simulink model "adcs_v15_integral_Power_dist"  (Simulink 7.4)
settings: Solver=ode4  StartTime=0.0  StopTime=120000  FixedStep=s_SIM_STEP_SIZE  RelTol=1e-3
values from neighbouring files (symbols this model uses):
  A = ((T_SIDE + .29)*1e-3)^2    [constants_v13.m]    (also in constants_v15.m; constants_v15_Pow.m; constants_v15_Pow_ss_error.m; constants_v16_integral_kartavya.m)
  AMP = 4e-8    (= 4e-08)    [constants_v15_Pow.m]
  Area_SP_S1 = 4*11*0.02025*0.04025    (= 0.03586275)    [constants_v15_Pow.m]    (also in constants_v15_Pow_ss_error.m; constants_v16_integral_light_sun_sgp_igrf_power_13Dec2011.m)
  Area_SP_S2 = 4*11*0.02025*0.04025    (= 0.03586275)    [constants_v15_Pow.m]    (also in constants_v15_Pow_ss_error.m; constants_v16_integral_light_sun_sgp_igrf_power_13Dec2011.m)
  Area_SP_S3 = 0.0    (= 0)    [constants_v15_Pow.m]    (also in constants_v15_Pow_ss_error.m; constants_v16_integral_light_sun_sgp_igrf_power_13Dec2011.m)
  Area_SP_S4 = 4*11*0.02025*0.04025    (= 0.03586275)    [constants_v15_Pow.m]    (also in constants_v15_Pow_ss_error.m; constants_v16_integral_light_sun_sgp_igrf_power_13Dec2011.m)
  Area_SP_S5 = 0.0    (= 0)    [constants_v15_Pow.m]    (also in constants_v15_Pow_ss_error.m; constants_v16_integral_light_sun_sgp_igrf_power_13Dec2011.m)
  Area_SP_S6 = 3*11*0.02025*0.04025    (= 0.0268970625)    [constants_v15_Pow.m]    (also in constants_v15_Pow_ss_error.m; constants_v16_integral_light_sun_sgp_igrf_power_13Dec2011.m)
  Ca_Solar_Drag = 1.4    [constants_v13.m]    (also in constants_v15.m; constants_v15_Pow.m; constants_v15_Pow_ss_error.m; constants_v16_integral_kartavya.m)
  Cd = 2.2    [constants_v13.m]    (also in constants_v15.m; constants_v15_Pow.m; constants_v15_Pow_ss_error.m; constants_v16_integral_kartavya.m)
  check_time = 60000    [constants_v13.m]    (also in constants_v15.m = 10000; constants_v15_Pow.m = 10000; constants_v15_Pow_ss_error.m = 10000; constants_v16_integral_kartavya.m = 10000)
  efficiany_solar_cell = 0.16    [constants_v15_Pow.m]    (also in constants_v15_Pow_ss_error.m; constants_v16_integral_light_sun_sgp_igrf_power_13Dec2011.m)
  equinox = datenum('21-Mar-2010 12:0:0')    [constants_v13.m]    (also in constants_v15.m; constants_v15_Pow.m; constants_v15_Pow_ss_error.m; constants_v16_integral_kartavya.m)
  I_MAX = 0.5    [constants_v13.m]    (also in constants_v15.m; constants_v15_Pow.m; constants_v15_Pow_ss_error.m; constants_v16_integral_kartavya.m)
  I_TORQUER = 3.6 / 7.31    (= 0.492476060192)    [constants_v13.m]    (also in constants_v15.m; constants_v15_Pow.m; constants_v15_Pow_ss_error.m; constants_v16_integral_kartavya.m)
  Kd = 2* m_INERTIA / (s_numOrbits * T_ORBIT )    [constants_v13.m]    (also in constants_v15.m = m_INERTIA * (2 + delta)* zeta * w; constants_v15_Pow.m = m_INERTIA * (2 + delta)* zeta * w; constants_v15_Pow_ss_error.m = m_INERTIA * (2 + delta)* zeta * w; constants_v16_integral_kartavya.m = m_INERTIA * (2 + delta)* zeta * w)
  Kdetumb = K_det*eye(3)    [constants_v13.m]    (also in constants_v15.m; constants_v15_Pow.m; constants_v15_Pow_ss_error.m; constants_v16_integral_kartavya.m)
  Ki = m_INERTIA * delta * zeta * w^3    [constants_v15.m]    (also in constants_v15_Pow.m; constants_v15_Pow_ss_error.m; constants_v16_integral_kartavya.m; constants_v16_integral_light_sun_sgp_igrf_power_13Dec2011.m)
  Kp = m_INERTIA / (s_numOrbits * T_ORBIT * zeta)^2    [constants_v13.m]    (also in constants_v15.m = m_INERTIA * (w*w + 2*delta*zeta^2*w^2); constants_v15_Pow.m = m_INERTIA * (w*w + 2*delta*zeta^2*w^2); constants_v15_Pow_ss_error.m = m_INERTIA * (w*w + 2*delta*zeta^2*w^2); constants_v16_integral_kartavya.m = m_INERTIA * (w*w + 2*delta*zeta^2*w^2))
  m_INERTIA = [Ixx Ixy Ixz; Ixy Iyy Iyz; Ixz Iyz Izz]    [constants_v13.m]    (also in constants_v15.m; constants_v15_Pow.m = 1*[Ixx Ixy Ixz; Ixy Iyy Iyz; Ixz Iyz Izz]; constants_v15_Pow_ss_error.m = 1*[Ixx Ixy Ixz; Ixy Iyy Iyz; Ixz Iyz Izz]; constants_v16_integral_kartavya.m)
  mu = 6.673e-11*5.9742e24    (= 398658366000000)    [constants_v13.m]    (also in constants_v15.m; constants_v15_Pow.m; constants_v15_Pow_ss_error.m; constants_v16_integral_kartavya.m)
  N = 40    [constants_v13.m]    (also in constants_v15.m; constants_v15_Pow.m; constants_v15_Pow_ss_error.m; constants_v16_integral_kartavya.m)
  P_momentum_flux_from_the_sun = 4.4e-6    (= 4.4e-06)    [constants_v13.m]    (also in constants_v15.m; constants_v15_Pow.m; constants_v15_Pow_ss_error.m; constants_v16_integral_kartavya.m)
  q_BI0 = euler2qBI(roll0,pitch0,yaw0)    [constants_v13.m]    (also in constants_v15.m; constants_v15_Pow.m; constants_v15_Pow_ss_error.m; constants_v16_integral_kartavya.m)
  s_FRAME_SIZE = 2    [constants_v13.m]    (also in constants_v15.m; constants_v15_Pow.m; constants_v15_Pow_ss_error.m; constants_v16_integral_kartavya.m)
  s_m_MAX = 0.95    [constants_v13.m]    (also in constants_v15.m; constants_v15_Pow.m; constants_v15_Pow_ss_error.m; constants_v16_integral_kartavya.m)
  s_MAG_B = 2.5e-5    (= 2.5e-05)    [constants_v13.m]    (also in constants_v15.m; constants_v15_Pow.m; constants_v15_Pow_ss_error.m; constants_v16_integral_kartavya.m)
  s_MAGMETER_WEIGHT = .9    (= 0.9)    [constants_v13.m]    (also in constants_v15.m; constants_v15_Pow.m; constants_v15_Pow_ss_error.m; constants_v16_integral_kartavya.m)
  s_SIM_STEP_SIZE = 0.1    [constants_v13.m]    (also in constants_v15.m; constants_v15_Pow.m; constants_v15_Pow_ss_error.m; constants_v16_integral_kartavya.m)
  s_SS_ADC_gain = 5    [constants_v13.m]    (also in constants_v15.m; constants_v15_Pow.m; constants_v15_Pow_ss_error.m; constants_v16_integral_kartavya.m)
  s_SS_ADC_res = 2^12 - 1    (= 4095)    [constants_v13.m]    (also in constants_v15.m; constants_v15_Pow.m; constants_v15_Pow_ss_error.m; constants_v16_integral_kartavya.m)
  s_SS_MAX_ANGLE = 85    [constants_v13.m]    (also in constants_v15.m; constants_v15_Pow.m; constants_v15_Pow_ss_error.m; constants_v16_integral_kartavya.m)
  s_TAU_W = 60    [constants_v13.m]    (also in constants_v15.m; constants_v15_Pow.m; constants_v15_Pow_ss_error.m; constants_v16_integral_kartavya.m)
  s_W_SAT = sqrt(mu/R_e^3)    [constants_v13.m]    (also in constants_v15.m; constants_v15_Pow.m; constants_v15_Pow_ss_error.m; constants_v16_integral_kartavya.m)
  s_x_MAGMETER_BIAS = 50e-9    (= 5e-08)    [constants_v13.m]    (also in constants_v15.m; constants_v15_Pow.m; constants_v15_Pow_ss_error.m; constants_v16_integral_kartavya.m)
  side = 0.26    [constants_v13.m]    (also in constants_v15.m; constants_v15_Pow.m; constants_v15_Pow_ss_error.m; constants_v16_integral_kartavya.m)
  Snum = 6    [constants_v13.m]    (also in constants_v15.m; constants_v15_Pow.m; constants_v15_Pow_ss_error.m; constants_v16_integral_kartavya.m)
  Solar_Constant = 1353    [constants_v15_Pow.m]    (also in constants_v15_Pow_ss_error.m; constants_v16_integral_light_sun_sgp_igrf_power_13Dec2011.m)
  today = datenum('18-Oct-2010 10:30:0')    [constants_v13.m]    (also in constants_v15.m; constants_v15_Pow.m; constants_v15_Pow_ss_error.m; constants_v16_integral_kartavya.m)
  tol_q4 = 0.7    [constants_v13.m]    (also in constants_v15.m = 0.85; constants_v15_Pow.m = 0.85; constants_v15_Pow_ss_error.m = 0.85; constants_v16_integral_kartavya.m = 0.85)
  tol_w = 4e-3    (= 0.004)    [constants_v13.m]    (also in constants_v15.m; constants_v15_Pow.m; constants_v15_Pow_ss_error.m; constants_v16_integral_kartavya.m)
  tolw_n2d = 10e-3    (= 0.01)    [constants_v15.m]    (also in constants_v15_Pow.m; constants_v15_Pow_ss_error.m; constants_v16_integral_kartavya.m; constants_v16_integral_light_sun_sgp_igrf_power_13Dec2011.m)
  Ts_display = 6    [constants_v13.m]    (also in constants_v15.m; constants_v15_Pow.m; constants_v15_Pow_ss_error.m; constants_v16_integral_kartavya.m)
  v_COM_to_COP_b = [.2; 1.75; .2]*1e-2    [constants_v13.m]    (also in constants_v15.m; constants_v15_Pow.m; constants_v15_Pow_ss_error.m; constants_v16_integral_kartavya.m)
  v_S1 = [1 0 0]    [constants_v13.m]    (also in constants_v15.m; constants_v15_Pow.m; constants_v15_Pow_ss_error.m; constants_v16_integral_kartavya.m)
  v_S2 = [-1 0 0]    [constants_v13.m]    (also in constants_v15.m; constants_v15_Pow.m; constants_v15_Pow_ss_error.m; constants_v16_integral_kartavya.m)
  v_S3 = [0 1 0]    [constants_v13.m]    (also in constants_v15.m; constants_v15_Pow.m; constants_v15_Pow_ss_error.m; constants_v16_integral_kartavya.m)
  v_S4 = [0 -1 0]    [constants_v13.m]    (also in constants_v15.m; constants_v15_Pow.m; constants_v15_Pow_ss_error.m; constants_v16_integral_kartavya.m)
  v_S5 = [0 0 1]    [constants_v13.m]    (also in constants_v15.m; constants_v15_Pow.m; constants_v15_Pow_ss_error.m; constants_v16_integral_kartavya.m)
  v_S6 = [0 0 -1]    [constants_v13.m]    (also in constants_v15.m; constants_v15_Pow.m; constants_v15_Pow_ss_error.m; constants_v16_integral_kartavya.m)
  v_x_MOUNTING_THETA_ZYX_BODY_TORQUER = [1; 1; 1]* pi/180    [constants_v13.m]    (also in constants_v15.m; constants_v15_Pow.m; constants_v15_Pow_ss_error.m; constants_v16_integral_kartavya.m)
  wx0 = 2*pi/180    (= 0.0349065850399)    [constants_v13.m]    (also in constants_v15.m = 0.00174532925199; constants_v15_Pow.m = 1.74532925199e-05; constants_v15_Pow_ss_error.m = 2.01533262693e-05; constants_v16_integral_kartavya.m = 0.0174532925199)
  wy0 = 1*pi/180    (= 0.0174532925199)    [constants_v13.m]    (also in constants_v15.m = 0.00174532925199; constants_v15_Pow.m = 1.74532925199e-05; constants_v15_Pow_ss_error.m = 2.01533262693e-05; constants_v16_integral_kartavya.m = 0)
  wz0 = -2*pi/180    (= -0.0349065850399)    [constants_v13.m]    (also in constants_v15.m = 0.00174532925199; constants_v15_Pow.m = 1.74532925199e-05; constants_v15_Pow_ss_error.m = 2.01533262693e-05; constants_v16_integral_kartavya.m = -0.00872664625997)
libraries: simulink x9, commnoisgen2 x7, aerolibutil x2
(part 1 of 2)
settings Model: Creator=Jaideep  LastModifiedBy=Ankit Shah  SimulationMode=rapid-accelerator  ExtModeTrigDuration=100
settings SolverCC: AutoInsertRateTranBlk=on
settings DataIOCC: ExternalInput=constants_v13  SaveFinalState=on  SaveOutput=off  SaveState=on  StateSaveName=tmp_raccel_xout
settings OptimizationCC: EfficientMapNaN2IntZero=off
settings HardwareCC: TargetEndianess=LittleEndian  TargetHWDeviceType=MATLAB Host  ProdEqTarget=off
settings RTWCC: SystemTargetFile=raccel.tlc  TemplateMakefile=raccel_default_tmf  RTWVerbose=off  ProcessScript=raccel_make_rtw_hook
settings CodeAppCC: GenerateComments=off  MaxIdLength=128  SimulinkBlockComments=off
settings RaccelTargetCC: TargetFunctionLibrary=ANSI_C  ERTMultiwordTypeDef=System defined  ERTMultiwordLength=256  IsPILTarget=off  ParMdlRefBuildCompliant=off  GeneratePreprocessorConditionals=Disable all  ERTFirstTimeCompliant=off  MultiInstanceERTCode=off  EnableShiftOperators=on  PortableWordSizes=off  RTWCAPISignals=off  RTWCAPIParams=off

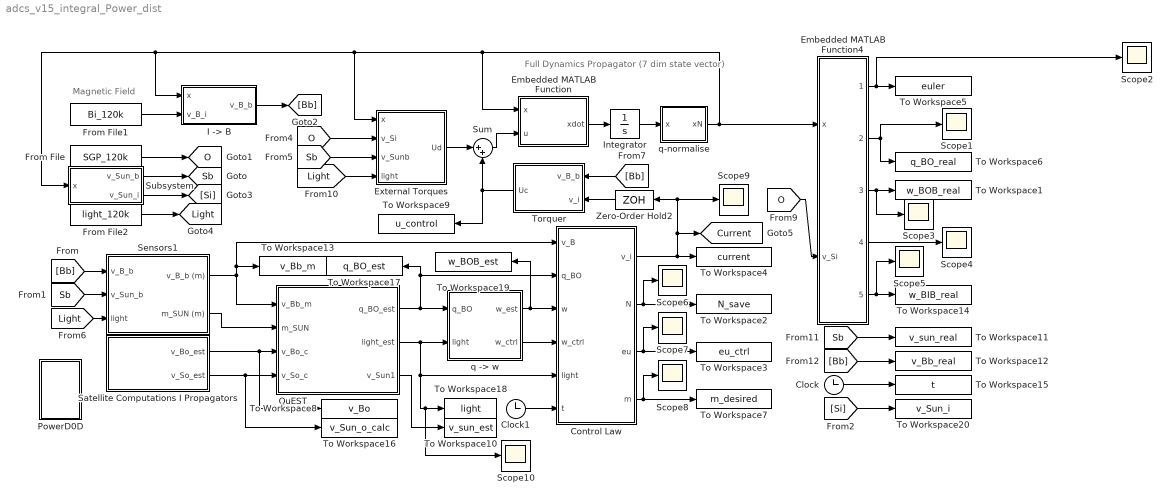
== system adcs_v15_integral_Power_dist ==
  note: Full Dynamics Propagator
      |  (7 dim state vector)
  note: Magnetic Field
  Clock : Clock
      settings: Decimation=10
  Clock1 : Clock
      settings: Decimation=10
  Control Law : Subsystem  TreatAsAtomicUnit=on  SystemSampleTime=s_FRAME_SIZE
  Embedded MATLAB Function : Stateflow chart  TreatAsAtomicUnit=on
  Embedded MATLAB Function4 : Stateflow chart  TreatAsAtomicUnit=on
  External Torques : Subsystem
  From File : FromFile  FileName=SGP_120k
  From File1 : FromFile  FileName=Bi_120k
  From File2 : FromFile  FileName=light_120k  SampleTime=0
  "I -> B" : Subsystem
  Integrator : Integrator  InitialCondition=[q_BI0; wx0; wy0; wz0]
  PowerD0D : Subsystem
  QuEST : Stateflow chart  TreatAsAtomicUnit=on  SystemSampleTime=s_FRAME_SIZE
  Satellite Computations I Propagators : Subsystem  TreatAsAtomicUnit=on  SystemSampleTime=s_FRAME_SIZE
  Scope{1..10} (10 alike) : Scope
      Scope1 settings: YMin=-0.1  YMax=1  SaveName=ScopeData11  SampleInput=on  SampleTime=Ts_display
      Scope10 settings: YMin=-10  YMax=10  SaveName=ScopeData3  SampleInput=on  SampleTime=Ts_display
      Scope2 settings: TimeRange=4.628195763325493  YMin=123.2676342903707  YMax=123.2853486115136  SaveName=ScopeData7  SampleInput=on  SampleTime=Ts_display
      Scope3 settings: YMin=-10  YMax=10  SaveName=ScopeData13  SampleInput=on  SampleTime=Ts_display
      Scope4 settings: YMin=7.5e-005  YMax=0.0006  SaveName=ScopeData14  SampleInput=on  SampleTime=Ts_display
      Scope5 settings: YMin=-10  YMax=10  SaveName=ScopeData15  SampleInput=on  SampleTime=Ts_display
      Scope6 settings: YMin=0  YMax=1  SaveName=ScopeData16  SampleInput=on  SampleTime=Ts_display
      Scope7 settings: YMin=-1  YMax=1  SaveName=ScopeData20  SampleInput=on  SampleTime=Ts_display
      Scope8 settings: YMin=-10  YMax=10  SaveName=ScopeData21  SampleInput=on  SampleTime=Ts_display
      Scope9 settings: YMin=-10  YMax=10  SaveName=ScopeData23  SampleInput=on  SampleTime=Ts_display
  Sensors1 : Subsystem
  Subsystem : Subsystem
  Sum : Sum  Inputs=|++  OutDataType=sfix(16)  OutScaling=2^0
  To Workspace1 : ToWorkspace  VariableName=w_BOB_real  SampleTime=Ts_display  SaveFormat=Array
  To Workspace10 : ToWorkspace  VariableName=v_sun_est  SampleTime=Ts_display  SaveFormat=Array
  To Workspace11 : ToWorkspace  VariableName=v_sun_real  SampleTime=Ts_display  SaveFormat=Array
  To Workspace12 : ToWorkspace  VariableName=v_Bb_real  SampleTime=Ts_display  SaveFormat=Array
  To Workspace13 : ToWorkspace  VariableName=v_Bb_m  SampleTime=Ts_display  SaveFormat=Array
  To Workspace14 : ToWorkspace  VariableName=w_BIB_real  SampleTime=Ts_display  SaveFormat=Array
  To Workspace15 : ToWorkspace  VariableName=t  SampleTime=Ts_display  SaveFormat=Array
  To Workspace16 : ToWorkspace  VariableName=v_Sun_o_calc  SampleTime=Ts_display  SaveFormat=Array
  To Workspace17 : ToWorkspace  VariableName=q_BO_est  SampleTime=Ts_display  SaveFormat=Array
  To Workspace18 : ToWorkspace  VariableName=light  SampleTime=Ts_display  SaveFormat=Array
  To Workspace19 : ToWorkspace  VariableName=w_BOB_est  SampleTime=Ts_display  SaveFormat=Array
  To Workspace2 : ToWorkspace  VariableName=N_save  SampleTime=Ts_display  SaveFormat=Array
  To Workspace20 : ToWorkspace  VariableName=v_Sun_i  SampleTime=Ts_display  SaveFormat=Array
  To Workspace3 : ToWorkspace  VariableName=eu_ctrl  SampleTime=Ts_display  SaveFormat=Array
  To Workspace4 : ToWorkspace  VariableName=current  SampleTime=Ts_display  SaveFormat=Array
  To Workspace5 : ToWorkspace  VariableName=euler  SampleTime=Ts_display  SaveFormat=Array
  To Workspace6 : ToWorkspace  VariableName=q_BO_real  SampleTime=Ts_display  SaveFormat=Array
  To Workspace7 : ToWorkspace  VariableName=m_desired  SampleTime=Ts_display  SaveFormat=Array
  To Workspace8 : ToWorkspace  VariableName=v_Bo  SampleTime=Ts_display  SaveFormat=Array
  To Workspace9 : ToWorkspace  VariableName=u_control  SampleTime=Ts_display  SaveFormat=Array
  Torquer : Subsystem
  Zero-Order Hold2 : ZeroOrderHold  SampleTime=s_FRAME_SIZE
  "q -> w" : Subsystem  TreatAsAtomicUnit=on  SystemSampleTime=s_FRAME_SIZE
  q-normalise : Stateflow chart  TreatAsAtomicUnit=on
  tag scope: Current=global, Light=global, O=global, Sb=global
  wires:
  Embedded MATLAB Function/1(xdot) -> Integrator/1
  Integrator/1 -> q-normalise/1(x)
  From File/1 -> [O]
  q-normalise/1(xN) -> Subsystem/1(x), "I -> B"/1(x), External Torques/1(x), Embedded MATLAB Function/1(x), Embedded MATLAB Function4/1(x)
  Sum/1 -> Embedded MATLAB Function/2(u)
  "I -> B"/1(v_B_b) -> [Bb]
  Subsystem/1(v_Sun_b) -> [Sb]
  [Bb] -> Sensors1/1(v_B_b)
  [Sb] -> Sensors1/2(v_Sun_b)
  Subsystem/2(v_Sun_i) -> [Si]
  [O] -> External Torques/2(v_Si)
  [Sb] -> External Torques/3(v_Sunb)
  [Bb] -> Torquer/1(v_B_b)
  [Light] -> Sensors1/3(light)
  Sensors1/2(m_SUN (m)) -> QuEST/2(m_SUN)
  Sensors1/1(v_B_b (m)) -> QuEST/1(v_Bb_m), Control Law/1(v_B), To Workspace13/1
  Zero-Order Hold2/1 -> Torquer/2(v_i)
  Torquer/1(Uc) -> Sum/2, To Workspace9/1
  Satellite Computations I Propagators/1(v_Bo_est) -> To Workspace8/1, QuEST/3(v_Bo_c)
  Satellite Computations I Propagators/2(v_So_est) -> To Workspace16/1, QuEST/4(v_So_c)
  QuEST/1(q_BO_est) -> "q -> w"/1(q_BO), Control Law/2(q_BO), To Workspace17/1
  QuEST/2(light_est) -> "q -> w"/2(light), Control Law/5(light), To Workspace18/1, Scope10/1
  Control Law/1(v_i) -> To Workspace4/1, Zero-Order Hold2/1, Scope9/1, [Current]
  [O] -> Embedded MATLAB Function4/2(v_Si)
  Control Law/2(N) -> To Workspace2/1, Scope6/1
  From File2/1 -> [Light]
  Control Law/3(eu) -> To Workspace3/1, Scope7/1
  Control Law/4(m) -> To Workspace7/1, Scope8/1
  "q -> w"/1(w_est) -> Control Law/3(w), To Workspace19/1
  [Light] -> External Torques/4(light)
  "q -> w"/2(w_ctrl) -> Control Law/4(w_ctrl)
  QuEST/3(v_Sun1) -> To Workspace10/1
  [Sb] -> To Workspace11/1
  [Bb] -> To Workspace12/1
  Clock/1 -> To Workspace15/1
  From File1/1 -> "I -> B"/2(v_B_i)
  Clock1/1 -> Control Law/6(t)
  Embedded MATLAB Function4/3(w_BOB) -> To Workspace1/1, Scope3/1
  Embedded MATLAB Function4/2(q_BO) -> To Workspace6/1, Scope1/1
  Embedded MATLAB Function4/1(euler) -> To Workspace5/1, Scope2/1
  Embedded MATLAB Function4/5(w_BIB) -> To Workspace14/1, Scope5/1
  Embedded MATLAB Function4/4(modw) -> Scope4/1
  [Si] -> To Workspace20/1
  External Torques/1(Ud) -> Sum/1

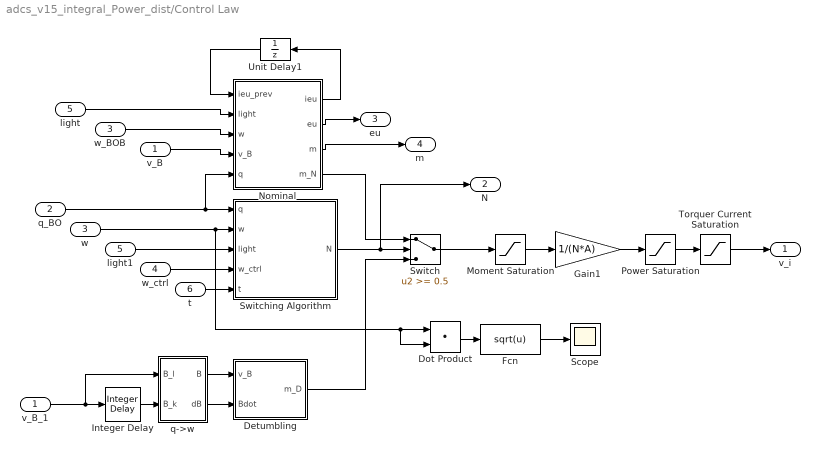
== system adcs_v15_integral_Power_dist/Control Law ==
  v_B : Inport  OutDataType=sfix(16)  OutScaling=2^0
  q_BO : Inport  Port=2  OutDataType=sfix(16)  OutScaling=2^0
  w : Inport  Port=3  OutDataType=sfix(16)  OutScaling=2^0
  w_ctrl : Inport  Port=4  OutDataType=sfix(16)  OutScaling=2^0
  light : Inport  Port=5  OutDataType=sfix(16)  OutScaling=2^0
  t : Inport  Port=6  OutDataType=sfix(16)  OutScaling=2^0
  Detumbling : Stateflow chart  TreatAsAtomicUnit=on
  Dot Product : DotProduct  OutDataType=fixdt(1, 16)  OutScaling=2^-10  InputSameDT=on  OutDataTypeStr=Inherit: Inherit via internal rule
  Fcn : Fcn  Expr=sqrt(u)
  Gain1 : Gain  Gain=1/(N*A)  ParameterDataType=sfix(16)  ParameterScaling=2^0  OutDataType=sfix(16)  OutScaling=2^0
  Integer Delay : simulink/Discrete/Integer Delay  vinit=0.0  samptime=-1  NumDelays=1
  Moment Saturation : Saturate  UpperLimit=s_m_MAX  LowerLimit=-s_m_MAX  OutDataType=sfix(16)  OutScaling=2^0
  Nominal : Stateflow chart  TreatAsAtomicUnit=on
  Power Saturation : Saturate  UpperLimit=I_MAX  LowerLimit=-I_MAX  OutDataType=sfix(16)  OutScaling=2^0
  Scope : Scope
      settings: YMin=0  YMax=0.11  SaveName=ScopeData4
  Switch : Switch  Threshold=0.5  OutDataType=sfix(16)  OutScaling=2^0
  Switching Algorithm : Subsystem
  Torquer Current Saturation : Saturate  UpperLimit=I_TORQUER  LowerLimit=-I_TORQUER  OutDataType=sfix(16)  OutScaling=2^0
  Unit Delay1 : UnitDelay  X0=[0;0;0]  SampleTime=-1
  light1 : InportShadow  Port=5  OutDataType=sfix(16)  OutScaling=2^0  LatchByCopyingInsideSignal=off
  q->w : Stateflow chart  TreatAsAtomicUnit=on
  v_B_1 : InportShadow  Port=1  OutDataType=sfix(16)  OutScaling=2^0  LatchByCopyingInsideSignal=off
  w_BOB : InportShadow  Port=3  OutDataType=sfix(16)  OutScaling=2^0  LatchByCopyingInsideSignal=off
  v_i : Outport  OutDataType=sfix(16)  OutScaling=2^0
  N : Outport  Port=2  OutDataType=sfix(16)  OutScaling=2^0
  eu : Outport  Port=3  OutDataType=sfix(16)  OutScaling=2^0
  m : Outport  Port=4  OutDataType=sfix(16)  OutScaling=2^0
  wires:
  w_ctrl/1 -> Switching Algorithm/4(w_ctrl)
  Nominal/3(m) -> m/1
  Nominal/2(eu) -> eu/1
  w_BOB/1 -> Nominal/3(w)
  light1/1 -> Switching Algorithm/3(light)
  v_B/1 -> Nominal/4(v_B)
  q->w/2(dB) -> Detumbling/2(Bdot)
  v_B_1/1 -> Integer Delay/1, q->w/1(B_l)
  w/1 -> Switching Algorithm/2(w), Dot Product/1, Dot Product/2
  Nominal/4(m_N) -> Switch/1
  Switching Algorithm/1(N) -> Switch/2, N/1
  Detumbling/1(m_D) -> Switch/3
  Switch/1 -> Moment Saturation/1
  Power Saturation/1 -> Torquer Current Saturation/1
  Moment Saturation/1 -> Gain1/1
  Torquer Current Saturation/1 -> v_i/1
  Gain1/1 -> Power Saturation/1
  light/1 -> Nominal/2(light)
  q_BO/1 -> Switching Algorithm/1(q), Nominal/5(q)
  Integer Delay/1 -> q->w/2(B_k)
  q->w/1(B) -> Detumbling/1(v_B)
  t/1 -> Switching Algorithm/5(t)
  Dot Product/1 -> Fcn/1
  Fcn/1 -> Scope/1
  Unit Delay1/1 -> Nominal/1(ieu_prev)
  Nominal/1(ieu) -> Unit Delay1/1

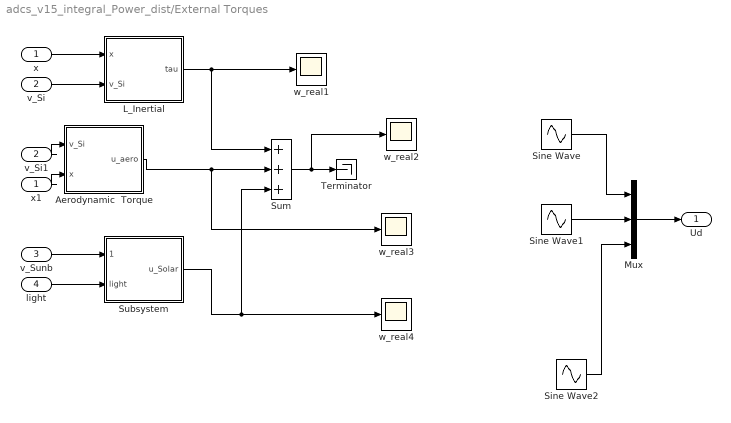
== system adcs_v15_integral_Power_dist/External Torques ==
  x : Inport  OutDataType=sfix(16)  OutScaling=2^0
  v_Si : Inport  Port=2  OutDataType=sfix(16)  OutScaling=2^0
  v_Sunb : Inport  Port=3  OutDataType=sfix(16)  OutScaling=2^0
  light : Inport  Port=4  OutDataType=sfix(16)  OutScaling=2^0
  Aerodynamic  Torque : Subsystem
  L_Inertial : Stateflow chart  TreatAsAtomicUnit=on
  Mux : Mux  Inputs=3
  Sine Wave : Sin  Amplitude=AMP  Bias=0  Frequency=2*s_W_SAT  Phase=0  Samples=10  SampleTime=0  Offset=0
  Sine Wave1 : Sin  Amplitude=AMP  Bias=0  Frequency=2*s_W_SAT  Phase=0  Samples=10  SampleTime=0  Offset=0
  Sine Wave2 : Sin  Amplitude=AMP  Bias=0  Frequency=2*s_W_SAT  Phase=0  Samples=10  SampleTime=0  Offset=0
  Subsystem : Subsystem
  Sum : Sum  Inputs=+++  OutDataType=fixdt(1, 16)  OutScaling=2^0
  Terminator : Terminator
  v_Si1 : InportShadow  Port=2  OutDataType=sfix(16)  OutScaling=2^0  LatchByCopyingInsideSignal=off
  w_real{1..4} (4 alike) : Scope
      w_real1 settings: TimeRange=80000  YMin=-3e-009  YMax=1.1e-008  SaveName=ScopeData18  SampleInput=on  SampleTime=5
      w_real2 settings: TimeRange=80000  YMin=-7e-009  YMax=1e-008  SaveName=ScopeData17  SampleInput=on  SampleTime=5
      w_real3 settings: YMin=-8e-010  YMax=1.4e-009  SaveName=ScopeData19  SampleInput=on  SampleTime=5
      w_real4 settings: YMin=-6e-009  YMax=1e-008  SaveName=ScopeData22  SampleInput=on  SampleTime=5
  x1 : InportShadow  Port=1  OutDataType=sfix(16)  OutScaling=2^0  LatchByCopyingInsideSignal=off
  Ud : Outport  OutDataType=sfix(16)  OutScaling=2^0
  wires:
  x/1 -> L_Inertial/1(x)
  v_Si/1 -> L_Inertial/2(v_Si)
  L_Inertial/1(tau) -> Sum/1, w_real1/1
  Aerodynamic  Torque/1(u_aero) -> Sum/2, w_real3/1
  x1/1 -> Aerodynamic  Torque/2(x)
  v_Si1/1 -> Aerodynamic  Torque/1(v_Si)
  Sum/1 -> w_real2/1, Terminator/1
  v_Sunb/1 -> Subsystem/1(v_Sun_b)
  Subsystem/1(u_Solar) -> Sum/3, w_real4/1
  light/1 -> Subsystem/2(light)
  Mux/1 -> Ud/1
  Sine Wave/1 -> Mux/1
  Sine Wave1/1 -> Mux/2
  Sine Wave2/1 -> Mux/3

== system adcs_v15_integral_Power_dist/I -> B ==
  x : Inport  OutDataType=sfix(16)  OutScaling=2^0
  v_B_i : Inport  Port=2  OutDataType=sfix(16)  OutScaling=2^0
  Gain : Gain  Gain=1e-9  ParameterDataType=fixdt(1, 16)  ParameterScaling=2^0  OutDataType=fixdt(1, 16)  OutScaling=2^0
  L_Inertial : Stateflow chart  TreatAsAtomicUnit=on
  v_B_b : Outport  OutDataType=sfix(16)  OutScaling=2^0
  wires:
  L_Inertial/1(v_B) -> v_B_b/1
  x/1 -> L_Inertial/1(x)
  v_B_i/1 -> Gain/1
  Gain/1 -> L_Inertial/2(v_I)

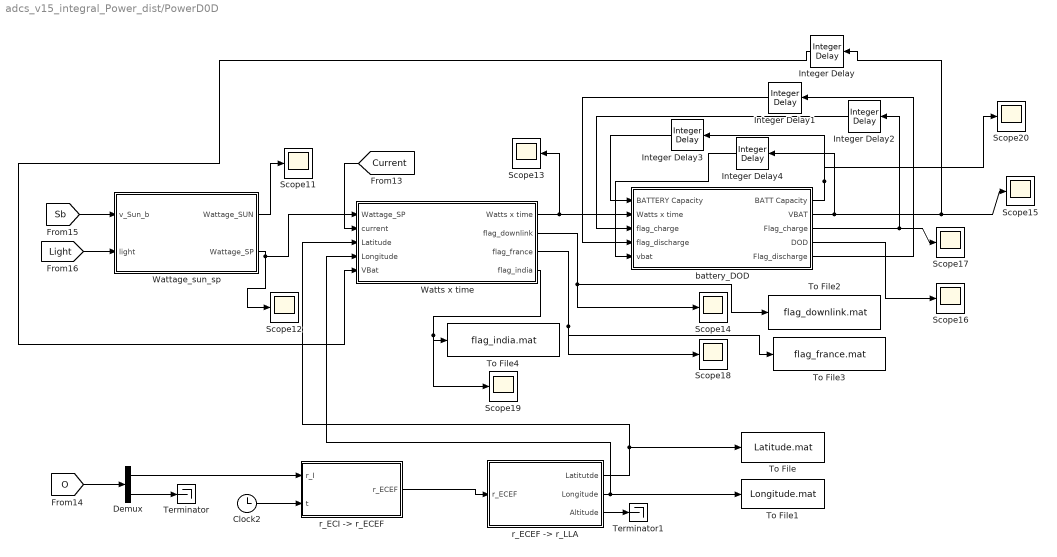
== system adcs_v15_integral_Power_dist/PowerD0D ==
  Clock2 : Clock
      settings: Decimation=10
  Demux : Demux  Outputs=2
  Integer Delay{,1..4} (5 alike) : simulink/Discrete/Integer Delay  vinit=0.0  samptime=-1  NumDelays=1
  Scope{11..20} (10 alike) : Scope
      Scope11 settings: YMin=0  YMax=47.5  SaveName=ScopeData29  SampleInput=on  SampleTime=Ts_display
      Scope12 settings: YMin=0  YMax=8  SaveName=ScopeData30  SampleInput=on  SampleTime=Ts_display
      Scope13 settings: YMin=-0.5  YMax=1.1  SaveName=ScopeData31  SampleInput=on  SampleTime=Ts_display
      Scope14 settings: YMin=0  YMax=1  SaveName=ScopeData25  SampleInput=on  SampleTime=Ts_display
      Scope15 settings: YMin=2.9  YMax=4.3  SaveName=ScopeData26  SampleInput=on  SampleTime=Ts_display
      Scope16 settings: YMin=0.898101  YMax=0.992637  SaveName=ScopeData27  SampleInput=on  SampleTime=Ts_display
      Scope17 settings: YMin=-60  SaveName=ScopeData28  SampleInput=on  SampleTime=Ts_display
      Scope18 settings: YMin=-1  YMax=1  SaveName=ScopeData32  SampleInput=on  SampleTime=Ts_display
      Scope19 settings: YMin=-1  YMax=1  SaveName=ScopeData33  SampleInput=on  SampleTime=Ts_display
      Scope20 settings: YMin=1000  YMax=2100  SaveName=ScopeData37  SampleInput=on  SampleTime=Ts_display
  Terminator : Terminator
  Terminator1 : Terminator
  To File : ToFile  Filename=Latitude.mat
  To File1 : ToFile  Filename=Longitude.mat
  To File2 : ToFile  Filename=flag_downlink.mat
  To File3 : ToFile  Filename=flag_france.mat
  To File4 : ToFile  Filename=flag_india.mat
  Wattage_sun_sp : Subsystem
  Watts x time : Subsystem
  battery_DOD : Subsystem
  "r_ECEF -> r_LLA" : Stateflow chart  TreatAsAtomicUnit=on
  "r_ECI -> r_ECEF" : Stateflow chart  TreatAsAtomicUnit=on
  wires:
  [Sb] -> Wattage_sun_sp/1(v_Sun_b)
  [Light] -> Wattage_sun_sp/2(light)
  Wattage_sun_sp/1(Wattage_SUN) -> Scope11/1
  Wattage_sun_sp/2(Wattage_SP) -> Scope12/1, Watts x time/1(Wattage_SP)
  [Current] -> Watts x time/2(current)
  battery_DOD/1(BATT Capacity) -> Scope20/1, Integer Delay3/1
  Integer Delay3/1 -> battery_DOD/1(BATTERY Capacity)
  [O] -> Demux/1
  Demux/2 -> Terminator/1
  Demux/1 -> "r_ECI -> r_ECEF"/1(r_I)
  Clock2/1 -> "r_ECI -> r_ECEF"/2(t)
  "r_ECI -> r_ECEF"/1(r_ECEF) -> "r_ECEF -> r_LLA"/1(r_ECEF)
  "r_ECEF -> r_LLA"/1(Latitutde) -> Watts x time/3(Latitude), To File/1
  "r_ECEF -> r_LLA"/2(Longitude) -> Watts x time/4(Longitude), To File1/1
  Watts x time/2(flag_downlink) -> Scope14/1, To File2/1
  battery_DOD/3(Flag_charge) -> Scope17/1, Integer Delay2/1
  Integer Delay2/1 -> battery_DOD/3(flag_charge)
  battery_DOD/2(VBAT) -> Scope15/1, Integer Delay/1, Integer Delay4/1
  battery_DOD/4(DOD) -> Scope16/1
  battery_DOD/5(Flag_discharge) -> Integer Delay1/1
  Integer Delay1/1 -> battery_DOD/4(flag_discharge)
  Integer Delay4/1 -> battery_DOD/5(vbat)
  Watts x time/3(flag_france) -> Scope18/1, To File3/1
  Watts x time/4(flag_india) -> To File4/1, Scope19/1
  Watts x time/1(Watts x time) -> battery_DOD/2(Watts x time), Scope13/1
  Integer Delay/1 -> Watts x time/5(VBat)
  "r_ECEF -> r_LLA"/3(Altitude) -> Terminator1/1

== system adcs_v15_integral_Power_dist/Satellite Computations I Propagators ==
  From File : FromFile  FileName=Si_120k
  From File2 : FromFile  FileName=SGP_est_120k
  From File3 : FromFile  FileName=Bi8_est_120k
  m_TOI_NEW : Stateflow chart  TreatAsAtomicUnit=on
  m_TOI_NEW1 : Stateflow chart  TreatAsAtomicUnit=on
  v_Bo_est : Outport  OutDataType=sfix(16)  OutScaling=2^0
  v_So_est : Outport  Port=2  OutDataType=sfix(16)  OutScaling=2^0
  wires:
  From File3/1 -> m_TOI_NEW/2(v_I)
  From File2/1 -> m_TOI_NEW1/2(ECI), m_TOI_NEW/1(ECI)
  From File/1 -> m_TOI_NEW1/1(v_I)
  m_TOI_NEW/1(v_O) -> v_Bo_est/1
  m_TOI_NEW1/1(v_O) -> v_So_est/1

== system adcs_v15_integral_Power_dist/Sensors1 ==
  note: 'm' stands for measured
  v_B_b : Inport  OutDataType=sfix(16)  OutScaling=2^0
  v_Sun_b : Inport  Port=2  OutDataType=sfix(16)  OutScaling=2^0
  light : Inport  Port=3  OutDataType=sfix(16)  OutScaling=2^0
  Magnetometer simple : Subsystem
  Sun Sensors : Subsystem
  v_B_b (m) : Outport  OutDataType=sfix(16)  OutScaling=2^0
  m_SUN (m) : Outport  Port=2  OutDataType=sfix(16)  OutScaling=2^0
  wires:
  light/1 -> Sun Sensors/2(Light)
  Magnetometer simple/1(v_B_b(m)) -> v_B_b (m)/1
  v_B_b/1 -> Magnetometer simple/1(v_B_b)
  v_Sun_b/1 -> Sun Sensors/1(v_Sun_b)
  Sun Sensors/1(m_SUN) -> m_SUN (m)/1

== system adcs_v15_integral_Power_dist/Subsystem ==
  x : Inport  OutDataType=sfix(16)  OutScaling=2^0
  From File : FromFile  FileName=Si_120k  SampleTime=0
  f: I->B : Stateflow chart  TreatAsAtomicUnit=on
  v_Sun_b : Outport  OutDataType=sfix(16)  OutScaling=2^0
  v_Sun_i : Outport  Port=2  OutDataType=sfix(16)  OutScaling=2^0
  wires:
  x/1 -> f: I->B/1(x)
  f: I->B/1(v_B) -> v_Sun_b/1
  From File/1 -> f: I->B/2(v_I), v_Sun_i/1

== system adcs_v15_integral_Power_dist/Torquer ==
  v_B_b : Inport  OutDataType=sfix(16)  OutScaling=2^0
  v_i : Inport  Port=2  OutDataType=sfix(16)  OutScaling=2^0
  3x3 Cross Product : aerolibutil/3x3 Cross Product  SystemSampleTime=-1
  Constant : Constant  Value=v_x_MOUNTING_THETA_ZYX_BODY_TORQUER  OutDataType=sfix(16)  OutScaling=2^0
  Embedded MATLAB Function4 : Stateflow chart  TreatAsAtomicUnit=on
  Gain : Gain  Gain=0  ParameterDataType=sfix(16)  ParameterScaling=2^0  OutDataType=sfix(16)  OutScaling=2^0
  Gain2 : Gain  Gain=N*A  ParameterDataType=sfix(16)  ParameterScaling=2^0  OutDataType=sfix(16)  OutScaling=2^0
  PWM : Quantizer  QuantizationInterval=s_PWM_RES
  Product : Product  Multiplication=Matrix(*)  OutDataType=sfix(16)  OutScaling=2^0  RndMeth=Zero
  Uc : Outport  OutDataType=sfix(16)  OutScaling=2^0
  wires:
  PWM/1 -> Gain2/1
  v_B_b/1 -> 3x3 Cross Product/2
  3x3 Cross Product/1 -> Uc/1
  v_i/1 -> PWM/1
  Embedded MATLAB Function4/1(DCM) -> Product/1
  Gain2/1 -> Product/2
  Product/1 -> 3x3 Cross Product/1
  Constant/1 -> Gain/1
  Gain/1 -> Embedded MATLAB Function4/1(euler)

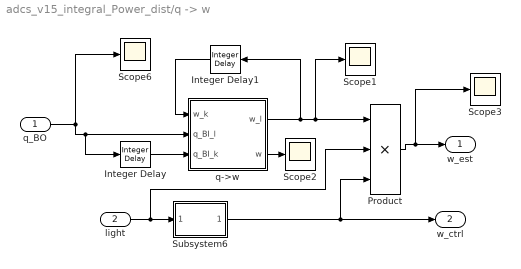
== system adcs_v15_integral_Power_dist/q -> w ==
  q_BO : Inport
  light : Inport  Port=2
  Integer Delay : simulink/Discrete/Integer Delay  vinit=0.0  samptime=-1  NumDelays=1
  Integer Delay1 : simulink/Discrete/Integer Delay  vinit=[0;0;0]  samptime=-1  NumDelays=1
  Product : Product  Inputs=3  OutDataType=fixdt(1, 16)  OutScaling=2^0  RndMeth=Zero
  Scope{1..3,6} (4 alike) : Scope
      Scope1 settings: YMin=-10  YMax=10  SaveName=ScopeData9  SampleInput=on
      Scope2 settings: YMin=-10  YMax=10  SaveName=ScopeData10  SampleInput=on
      Scope3 settings: YMin=-10  YMax=10  SaveName=ScopeData12  SampleInput=on
      Scope6 settings: YMin=-10  YMax=10  SaveName=ScopeData8  SampleInput=on
  Subsystem6 : Subsystem
  q->w : Stateflow chart  TreatAsAtomicUnit=on
  w_est : Outport
  w_ctrl : Outport  Port=2
  wires:
  Subsystem6/1(w-ctrl) -> w_ctrl/1, Product/3
  q_BO/1 -> Integer Delay/1, q->w/2(q_BI_l), Scope6/1
  light/1 -> Product/2, Subsystem6/1(light)
  Product/1 -> w_est/1, Scope3/1
  Integer Delay/1 -> q->w/3(q_BI_k)
  q->w/1(w_l) -> Integer Delay1/1, Product/1, Scope1/1
  Integer Delay1/1 -> q->w/1(w_k)
  q->w/2(w) -> Scope2/1

== system adcs_v15_integral_Power_dist/Control Law/Switching Algorithm ==
  note: remov the t=0 checking
      | code, not necessary
  q : Inport  OutDataType=sfix(16)  OutScaling=2^0
  w : Inport  Port=2  OutDataType=sfix(16)  OutScaling=2^0
  light : Inport  Port=3  OutDataType=sfix(16)  OutScaling=2^0
  w_ctrl : Inport  Port=4  OutDataType=sfix(16)  OutScaling=2^0
  t : Inport  Port=5  OutDataType=sfix(16)  OutScaling=2^0
  Scope1 : Scope
      settings: TimeRange=140000  YMin=0  YMax=1.3  SaveName=ScopeData5
  Unit Delay : UnitDelay  SampleTime=-1
  Unit Delay1 : UnitDelay  SampleTime=-1
  gate pulse : Stateflow chart  TreatAsAtomicUnit=on
  N : Outport  OutDataType=sfix(16)  OutScaling=2^0
  wires:
  t/1 -> gate pulse/4(t)
  w_ctrl/1 -> gate pulse/6(w_ctrl)
  light/1 -> gate pulse/5(light_flag)
  gate pulse/1(N) -> N/1, Unit Delay1/1
  q/1 -> gate pulse/3(q)
  gate pulse/3(t_now) -> Unit Delay/1
  w/1 -> gate pulse/2(w)
  Unit Delay/1 -> gate pulse/7(t_now_prev)
  Unit Delay1/1 -> gate pulse/1(N_prev)
  gate pulse/2(P) -> Scope1/1

== system adcs_v15_integral_Power_dist/External Torques/Aerodynamic  Torque ==
  v_Si : Inport
  x : Inport  Port=2
  Constant : Constant  Value=1e-14  OutDataType=fixdt(1, 16)  OutScaling=2^0
  Demux : Demux  Outputs=2
  aero torque : Stateflow chart  TreatAsAtomicUnit=on
  v_I to v_B : Stateflow chart  TreatAsAtomicUnit=on
  u_aero : Outport  OutDataType=sfix(16)  OutScaling=2^0
  wires:
  v_I to v_B/1(v_B) -> aero torque/2(v_B)
  v_Si/1 -> Demux/1
  Demux/2 -> v_I to v_B/1(v_I)
  x/1 -> v_I to v_B/2(x)
  aero torque/1(u_aero) -> u_aero/1
  Constant/1 -> aero torque/1(rho)

== system adcs_v15_integral_Power_dist/External Torques/Subsystem ==
  v_Sun_b : Inport  OutDataType=sfix(16)  OutScaling=2^0
  light : Inport  Port=2  OutDataType=sfix(16)  OutScaling=2^0
  Solar_drag : Stateflow chart  TreatAsAtomicUnit=on
  Vector from CoM to CoP_in Body frame (yet to be finalized)2 : Constant  Value=v_COM_to_COP_b  VectorParams1D=off  OutDataType=sfix(16)  OutScaling=2^0
  _ : aerolibutil/3x3 Cross Product  SystemSampleTime=-1
  u_Solar : Outport  OutDataType=sfix(16)  OutScaling=2^0
  wires:
  _/1 -> u_Solar/1
  v_Sun_b/1 -> Solar_drag/1(v_Sun_b)
  light/1 -> Solar_drag/2(light)
  Solar_drag/1(solar_drag) -> _/2
  Vector from CoM to CoP_in Body frame (yet to be finalized)2/1 -> _/1

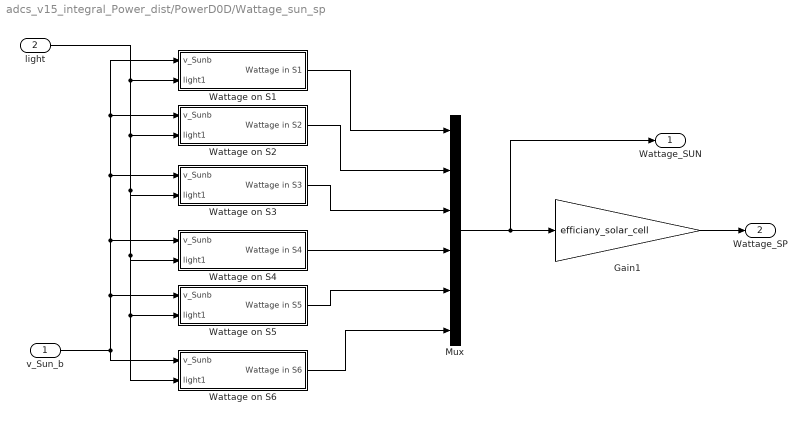
== system adcs_v15_integral_Power_dist/PowerD0D/Wattage_sun_sp ==
  v_Sun_b : Inport  OutDataType=sfix(16)  OutScaling=2^0
  light : Inport  Port=2  OutDataType=sfix(16)  OutScaling=2^0
  Gain1 : Gain  Gain=efficiany_solar_cell  ParameterDataType=sfix(16)  ParameterScaling=2^0  OutDataType=sfix(16)  OutScaling=2^0
  Mux : Mux  Inputs=6
  Wattage on S1 : Subsystem
  Wattage on S2 : Subsystem
  Wattage on S3 : Subsystem
  Wattage on S4 : Subsystem
  Wattage on S5 : Subsystem
  Wattage on S6 : Subsystem
  Wattage_SUN : Outport  OutDataType=fixdt(1, 16)  OutScaling=2^0
  Wattage_SP : Outport  Port=2  OutDataType=fixdt(1, 16)  OutScaling=2^0
  wires:
  v_Sun_b/1 -> Wattage on S6/1(v_Sunb), Wattage on S1/1(v_Sunb), Wattage on S2/1(v_Sunb), Wattage on S3/1(v_Sunb), Wattage on S4/1(v_Sunb), Wattage on S5/1(v_Sunb)
  light/1 -> Wattage on S1/2(light1), Wattage on S2/2(light1), Wattage on S3/2(light1), Wattage on S4/2(light1), Wattage on S5/2(light1), Wattage on S6/2(light1)
  Mux/1 -> Wattage_SUN/1, Gain1/1
  Gain1/1 -> Wattage_SP/1
  Wattage on S1/1(Wattage in S1) -> Mux/1
  Wattage on S2/1(Wattage in S2) -> Mux/2
  Wattage on S3/1(Wattage in S3) -> Mux/3
  Wattage on S4/1(Wattage in S4) -> Mux/4
  Wattage on S5/1(Wattage in S5) -> Mux/5
  Wattage on S6/1(Wattage in S6) -> Mux/6

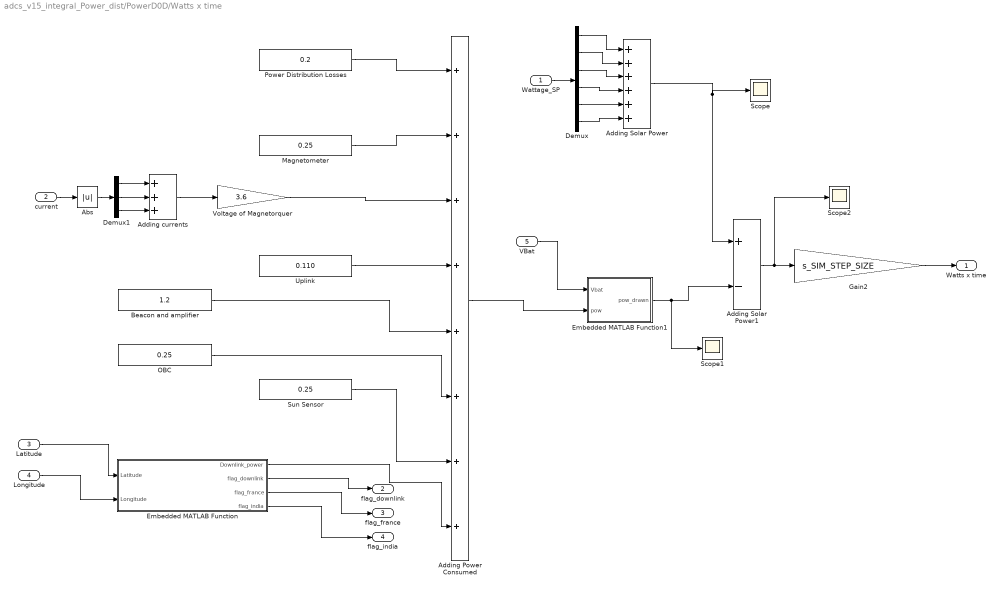
== system adcs_v15_integral_Power_dist/PowerD0D/Watts x time ==
  Wattage_SP : Inport  OutDataType=sfix(16)  OutScaling=2^0
  current : Inport  Port=2  OutDataType=sfix(16)  OutScaling=2^0
  Latitude : Inport  Port=3  OutDataType=sfix(16)  OutScaling=2^0
  Longitude : Inport  Port=4  OutDataType=sfix(16)  OutScaling=2^0
  VBat : Inport  Port=5  OutDataType=sfix(16)  OutScaling=2^0
  Abs : Abs  OutDataType=fixdt(1, 16)  OutScaling=2^0
  Adding Power Consumed : Sum  Inputs=++++++++  OutDataType=fixdt(1, 16)  OutScaling=2^-10
  Adding Solar Power : Sum  Inputs=++++++  OutDataType=fixdt(1, 16)  OutScaling=2^-10
  Adding Solar Power1 : Sum  Inputs=+-  OutDataType=fixdt(1, 16)  OutScaling=2^-10
  Adding currents : Sum  Inputs=+++  OutDataType=fixdt(1, 16)  OutScaling=2^-10
  Beacon and amplifier : Constant  Value=1.2  OutDataType=fixdt(1, 16)  OutScaling=2^0
  Demux : Demux  Outputs=6
  Demux1 : Demux  Outputs=3
  Embedded MATLAB Function : Stateflow chart  TreatAsAtomicUnit=on
  Embedded MATLAB Function1 : Stateflow chart  TreatAsAtomicUnit=on
  Gain2 : Gain  Gain=s_SIM_STEP_SIZE  ParameterDataType=fixdt(1, 16)  ParameterScaling=2^0  OutDataType=fixdt(1, 16)  OutScaling=2^0
  Magnetometer : Constant  Value=0.25  OutDataType=fixdt(1, 16)  OutScaling=2^0
  OBC : Constant  Value=0.25  OutDataType=fixdt(1, 16)  OutScaling=2^0
  Power Distribution Losses : Constant  Value=0.2  OutDataType=fixdt(1, 16)  OutScaling=2^0
  Scope : Scope
      settings: YMin=0  YMax=10.5  SaveName=ScopeData34
  Scope1 : Scope
      settings: YMin=2.25  SaveName=ScopeData35
  Scope2 : Scope
      settings: YMin=6.275  YMax=6.8  SaveName=ScopeData36
  Sun Sensor : Constant  Value=0.25  OutDataType=fixdt(1, 16)  OutScaling=2^0
  Uplink : Constant  Value=0.110  OutDataType=fixdt(1, 16)  OutScaling=2^0
  Voltage of Magnetorquer : Gain  Gain=3.6  ParameterDataType=fixdt(1, 16)  ParameterScaling=2^0  OutDataType=fixdt(1, 16)  OutScaling=2^0
  Watts x time : Outport  OutDataType=fixdt(1, 16)  OutScaling=2^0
  flag_downlink : Outport  Port=2  OutDataType=fixdt(1, 16)  OutScaling=2^0
  flag_france : Outport  Port=3  OutDataType=fixdt(1, 16)  OutScaling=2^0
  flag_india : Outport  Port=4  OutDataType=fixdt(1, 16)  OutScaling=2^0
  wires:
  Wattage_SP/1 -> Demux/1
  Demux/1 -> Adding Solar Power/1
  Demux/2 -> Adding Solar Power/2
  current/1 -> Abs/1
  Abs/1 -> Demux1/1
  Demux1/1 -> Adding currents/1
  Demux1/2 -> Adding currents/2
  Demux1/3 -> Adding currents/3
  Adding currents/1 -> Voltage of Magnetorquer/1
  Gain2/1 -> Watts x time/1
  Latitude/1 -> Embedded MATLAB Function/1(Latitude)
  Longitude/1 -> Embedded MATLAB Function/2(Longitude)
  Embedded MATLAB Function/2(flag_downlink) -> flag_downlink/1
  Embedded MATLAB Function/3(flag_france) -> flag_france/1
  Embedded MATLAB Function/4(flag_india) -> flag_india/1
  Power Distribution Losses/1 -> Adding Power Consumed/1
  Magnetometer/1 -> Adding Power Consumed/2
  Voltage of Magnetorquer/1 -> Adding Power Consumed/3
  Uplink/1 -> Adding Power Consumed/4
  Beacon and amplifier/1 -> Adding Power Consumed/5
  OBC/1 -> Adding Power Consumed/6
  Sun Sensor/1 -> Adding Power Consumed/7
  Embedded MATLAB Function/1(Downlink_power) -> Adding Power Consumed/8
  Demux/3 -> Adding Solar Power/3
  Demux/4 -> Adding Solar Power/4
  Demux/5 -> Adding Solar Power/5
  Demux/6 -> Adding Solar Power/6
  Adding Solar Power/1 -> Adding Solar Power1/1, Scope/1
  Adding Solar Power1/1 -> Gain2/1, Scope2/1
  VBat/1 -> Embedded MATLAB Function1/1(Vbat)
  Adding Power Consumed/1 -> Embedded MATLAB Function1/2(pow)
  Embedded MATLAB Function1/1(pow_drawn) -> Adding Solar Power1/2, Scope1/1

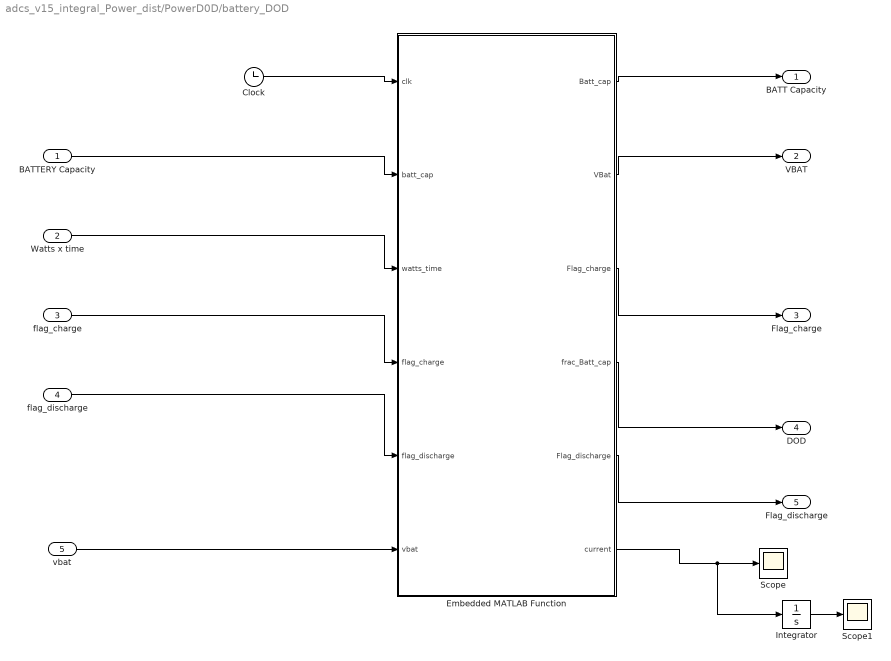
== system adcs_v15_integral_Power_dist/PowerD0D/battery_DOD ==
  BATTERY Capacity : Inport  OutDataType=sfix(16)  OutScaling=2^0
  Watts x time : Inport  Port=2  OutDataType=sfix(16)  OutScaling=2^0
  flag_charge : Inport  Port=3  OutDataType=sfix(16)  OutScaling=2^0
  flag_discharge : Inport  Port=4  OutDataType=sfix(16)  OutScaling=2^0
  vbat : Inport  Port=5  OutDataType=sfix(16)  OutScaling=2^0
  Clock : Clock
      settings: Decimation=10
  Embedded MATLAB Function : Stateflow chart  TreatAsAtomicUnit=on
  Integrator : Integrator
  Scope : Scope
      settings: YMin=-0.625  YMax=-0.275  SaveName=ScopeData38
  Scope1 : Scope
      settings: YMin=-0.625  YMax=-0.275  SaveName=ScopeData39
  BATT Capacity : Outport  OutDataType=fixdt(1, 16)  OutScaling=2^0
  VBAT : Outport  Port=2  OutDataType=fixdt(1, 16)  OutScaling=2^0
  Flag_charge : Outport  Port=3  OutDataType=fixdt(1, 16)  OutScaling=2^0
  DOD : Outport  Port=4  OutDataType=fixdt(1, 16)  OutScaling=2^0
  Flag_discharge : Outport  Port=5  OutDataType=fixdt(1, 16)  OutScaling=2^0
  wires:
  Clock/1 -> Embedded MATLAB Function/1(clk)
  BATTERY Capacity/1 -> Embedded MATLAB Function/2(batt_cap)
  Embedded MATLAB Function/1(Batt_cap) -> BATT Capacity/1
  Embedded MATLAB Function/2(VBat) -> VBAT/1
  Embedded MATLAB Function/3(Flag_charge) -> Flag_charge/1
  Watts x time/1 -> Embedded MATLAB Function/3(watts_time)
  flag_charge/1 -> Embedded MATLAB Function/4(flag_charge)
  Embedded MATLAB Function/4(frac_Batt_cap) -> DOD/1
  flag_discharge/1 -> Embedded MATLAB Function/5(flag_discharge)
  Embedded MATLAB Function/5(Flag_discharge) -> Flag_discharge/1
  vbat/1 -> Embedded MATLAB Function/6(vbat)
  Embedded MATLAB Function/6(current) -> Scope/1, Integrator/1
  Integrator/1 -> Scope1/1

== system adcs_v15_integral_Power_dist/Sensors1/Magnetometer simple ==
  v_B_b : Inport  OutDataType=sfix(16)  OutScaling=2^0
  Constant : Constant  Value=s_x_MAGMETER_BIAS  OutDataType=fixdt(1, 16)  OutScaling=2^0
  Gaussian Noise Generator : commnoisgen2/Gaussian Noise Generator  SystemSampleTime=-1  m=0  d=s_x_MAGMETER  s=41  Ts=s_SIM_STEP_SIZE  frameBased=off  sampPerFrame=1  orient=off  outDataType=double
  Sum1 : Sum  Inputs=+++  OutDataType=sfix(16)  OutScaling=2^0
  v_B_b(m) : Outport  OutDataType=sfix(16)  OutScaling=2^0
  wires:
  Constant/1 -> Sum1/3
  Sum1/1 -> v_B_b(m)/1
  Gaussian Noise Generator/1 -> Sum1/1
  v_B_b/1 -> Sum1/2

== system adcs_v15_integral_Power_dist/Sensors1/Sun Sensors ==
  v_Sun_b : Inport  OutDataType=sfix(16)  OutScaling=2^0
  Light : Inport  Port=2  OutDataType=sfix(16)  OutScaling=2^0
  Embedded MATLAB Function : Stateflow chart  TreatAsAtomicUnit=on
  S1 : Subsystem
  S2 : Subsystem
  S3 : Subsystem
  S4 : Subsystem
  S5 : Subsystem
  S6 : Subsystem
  m_SUN : Outport  OutDataType=fixdt(1, 16)  OutScaling=2^0
  wires:
  Embedded MATLAB Function/1(m_SUN) -> m_SUN/1
  v_Sun_b/1 -> S6/2(v_Sunb), S5/2(v_Sunb), S4/2(v_Sunb), S3/2(v_Sunb), S2/2(v_Sunb), S1/2(v_Sunb)
  S1/1(v_S) -> Embedded MATLAB Function/1(v_S1)
  S1/2(s_S) -> Embedded MATLAB Function/2(s_S1)
  S2/1(v_S) -> Embedded MATLAB Function/3(v_S2)
  S2/2(s_S) -> Embedded MATLAB Function/4(s_S2)
  S3/1(v_S) -> Embedded MATLAB Function/5(v_S3)
  S3/2(s_S) -> Embedded MATLAB Function/6(s_S3)
  S4/1(v_S) -> Embedded MATLAB Function/7(v_S4)
  S4/2(s_S) -> Embedded MATLAB Function/8(s_S4)
  S5/1(v_S) -> Embedded MATLAB Function/9(v_S5)
  S5/2(s_S) -> Embedded MATLAB Function/10(s_S5)
  S6/1(v_S) -> Embedded MATLAB Function/11(v_S6)
  S6/2(s_S) -> Embedded MATLAB Function/12(s_S6)
  Light/1 -> S1/1(light), S2/1(light), S3/1(light), S4/1(light), S5/1(light), S6/1(light)

== system adcs_v15_integral_Power_dist/q -> w/Subsystem6 ==
  light : Inport  OutDataType=fixdt(1, 16)  OutScaling=2^0
  (1-L) + L/z : Stateflow chart  TreatAsAtomicUnit=on
  Integer Delay : simulink/Discrete/Integer Delay  vinit=0.0  samptime=-1  NumDelays=300
  Scope : Scope
  Scope1 : Scope
  Scope2 : Scope
      settings: TimeRange=80000  SaveName=ScopeData2
  w-ctrl : Outport  OutDataType=fixdt(1, 16)  OutScaling=2^0
  wires:
  (1-L) + L/z/1(y) -> Scope/1, w-ctrl/1
  light/1 -> (1-L) + L/z/1(a), Integer Delay/1, Scope2/1
  Integer Delay/1 -> Scope1/1, (1-L) + L/z/2(b)

== system adcs_v15_integral_Power_dist/PowerD0D/Wattage_sun_sp/Wattage on S1 ==
  v_Sunb : Inport  OutDataType=sfix(16)  OutScaling=2^0
  light1 : Inport  Port=2  OutDataType=sfix(16)  OutScaling=2^0
  Constant : Constant  Value=v_S1  OutDataType=sfix(16)  OutScaling=2^0
  Dot Product : DotProduct  OutDataType=sfix(16)  OutScaling=2^-10  InputSameDT=on  OutDataTypeStr=Inherit: Inherit via internal rule
  Gain : Gain  Gain=Solar_Constant  ParameterDataType=sfix(16)  ParameterScaling=2^0  OutDataType=sfix(16)  OutScaling=2^0
  Gain1 : Gain  Gain=Area_SP_S1  ParameterDataType=sfix(16)  ParameterScaling=2^0  OutDataType=sfix(16)  OutScaling=2^0
  Product1 : Product  OutDataType=fixdt(1, 16)  OutScaling=2^0  RndMeth=Zero
  Saturation : Saturate  UpperLimit=1000  LowerLimit=0  OutDataType=fixdt(1, 16)  OutScaling=2^0
  Wattage in S1 : Outport  OutDataType=sfix(16)  OutScaling=2^0
  wires:
  v_Sunb/1 -> Dot Product/2
  Constant/1 -> Dot Product/1
  Gain1/1 -> Gain/1
  Gain/1 -> Wattage in S1/1
  Dot Product/1 -> Product1/1
  light1/1 -> Product1/2
  Product1/1 -> Saturation/1
  Saturation/1 -> Gain1/1

== system adcs_v15_integral_Power_dist/PowerD0D/Wattage_sun_sp/Wattage on S2 ==
  v_Sunb : Inport  OutDataType=sfix(16)  OutScaling=2^0
  light1 : Inport  Port=2  OutDataType=sfix(16)  OutScaling=2^0
  Constant : Constant  Value=v_S2  OutDataType=sfix(16)  OutScaling=2^0
  Dot Product : DotProduct  OutDataType=sfix(16)  OutScaling=2^-10  InputSameDT=on  OutDataTypeStr=Inherit: Inherit via internal rule
  Gain : Gain  Gain=Solar_Constant  ParameterDataType=sfix(16)  ParameterScaling=2^0  OutDataType=sfix(16)  OutScaling=2^0
  Gain1 : Gain  Gain=Area_SP_S2  ParameterDataType=sfix(16)  ParameterScaling=2^0  OutDataType=sfix(16)  OutScaling=2^0
  Product1 : Product  OutDataType=fixdt(1, 16)  OutScaling=2^0  RndMeth=Zero
  Saturation : Saturate  UpperLimit=1000  LowerLimit=0  OutDataType=fixdt(1, 16)  OutScaling=2^0
  Wattage in S2 : Outport  OutDataType=sfix(16)  OutScaling=2^0
  wires:
  v_Sunb/1 -> Dot Product/2
  Constant/1 -> Dot Product/1
  Gain1/1 -> Gain/1
  Gain/1 -> Wattage in S2/1
  Dot Product/1 -> Product1/1
  light1/1 -> Product1/2
  Product1/1 -> Saturation/1
  Saturation/1 -> Gain1/1

== system adcs_v15_integral_Power_dist/PowerD0D/Wattage_sun_sp/Wattage on S3 ==
  v_Sunb : Inport  OutDataType=sfix(16)  OutScaling=2^0
  light1 : Inport  Port=2  OutDataType=sfix(16)  OutScaling=2^0
  Constant : Constant  Value=v_S3  OutDataType=sfix(16)  OutScaling=2^0
  Dot Product : DotProduct  OutDataType=sfix(16)  OutScaling=2^-10  InputSameDT=on  OutDataTypeStr=Inherit: Inherit via internal rule
  Gain : Gain  Gain=Solar_Constant  ParameterDataType=sfix(16)  ParameterScaling=2^0  OutDataType=sfix(16)  OutScaling=2^0
  Gain1 : Gain  Gain=Area_SP_S3  ParameterDataType=sfix(16)  ParameterScaling=2^0  OutDataType=sfix(16)  OutScaling=2^0
  Product1 : Product  OutDataType=fixdt(1, 16)  OutScaling=2^0  RndMeth=Zero
  Saturation : Saturate  UpperLimit=1000  LowerLimit=0  OutDataType=fixdt(1, 16)  OutScaling=2^0
  Wattage in S3 : Outport  OutDataType=sfix(16)  OutScaling=2^0
  wires:
  v_Sunb/1 -> Dot Product/2
  Constant/1 -> Dot Product/1
  Gain1/1 -> Gain/1
  Gain/1 -> Wattage in S3/1
  Dot Product/1 -> Product1/1
  light1/1 -> Product1/2
  Product1/1 -> Saturation/1
  Saturation/1 -> Gain1/1

== system adcs_v15_integral_Power_dist/PowerD0D/Wattage_sun_sp/Wattage on S4 ==
  v_Sunb : Inport  OutDataType=sfix(16)  OutScaling=2^0
  light1 : Inport  Port=2  OutDataType=sfix(16)  OutScaling=2^0
  Constant : Constant  Value=v_S4  OutDataType=sfix(16)  OutScaling=2^0
  Dot Product : DotProduct  OutDataType=sfix(16)  OutScaling=2^-10  InputSameDT=on  OutDataTypeStr=Inherit: Inherit via internal rule
  Gain : Gain  Gain=Solar_Constant  ParameterDataType=sfix(16)  ParameterScaling=2^0  OutDataType=sfix(16)  OutScaling=2^0
  Gain1 : Gain  Gain=Area_SP_S4  ParameterDataType=sfix(16)  ParameterScaling=2^0  OutDataType=sfix(16)  OutScaling=2^0
  Product1 : Product  OutDataType=fixdt(1, 16)  OutScaling=2^0  RndMeth=Zero
  Saturation : Saturate  UpperLimit=1000  LowerLimit=0  OutDataType=fixdt(1, 16)  OutScaling=2^0
  Wattage in S4 : Outport  OutDataType=sfix(16)  OutScaling=2^0
  wires:
  v_Sunb/1 -> Dot Product/2
  Constant/1 -> Dot Product/1
  Gain1/1 -> Gain/1
  Gain/1 -> Wattage in S4/1
  Dot Product/1 -> Product1/1
  light1/1 -> Product1/2
  Product1/1 -> Saturation/1
  Saturation/1 -> Gain1/1

== system adcs_v15_integral_Power_dist/PowerD0D/Wattage_sun_sp/Wattage on S5 ==
  v_Sunb : Inport  OutDataType=sfix(16)  OutScaling=2^0
  light1 : Inport  Port=2  OutDataType=sfix(16)  OutScaling=2^0
  Constant : Constant  Value=v_S5  OutDataType=sfix(16)  OutScaling=2^0
  Dot Product : DotProduct  OutDataType=sfix(16)  OutScaling=2^-10  InputSameDT=on  OutDataTypeStr=Inherit: Inherit via internal rule
  Gain : Gain  Gain=Solar_Constant  ParameterDataType=sfix(16)  ParameterScaling=2^0  OutDataType=sfix(16)  OutScaling=2^0
  Gain1 : Gain  Gain=Area_SP_S5  ParameterDataType=sfix(16)  ParameterScaling=2^0  OutDataType=sfix(16)  OutScaling=2^0
  Product1 : Product  OutDataType=fixdt(1, 16)  OutScaling=2^0  RndMeth=Zero
  Saturation : Saturate  UpperLimit=1000  LowerLimit=0  OutDataType=fixdt(1, 16)  OutScaling=2^0
  Wattage in S5 : Outport  OutDataType=sfix(16)  OutScaling=2^0
  wires:
  v_Sunb/1 -> Dot Product/2
  Constant/1 -> Dot Product/1
  Gain1/1 -> Gain/1
  Gain/1 -> Wattage in S5/1
  Dot Product/1 -> Product1/1
  light1/1 -> Product1/2
  Product1/1 -> Saturation/1
  Saturation/1 -> Gain1/1

== system adcs_v15_integral_Power_dist/PowerD0D/Wattage_sun_sp/Wattage on S6 ==
  v_Sunb : Inport  OutDataType=sfix(16)  OutScaling=2^0
  light1 : Inport  Port=2  OutDataType=sfix(16)  OutScaling=2^0
  Constant : Constant  Value=v_S6  OutDataType=sfix(16)  OutScaling=2^0
  Dot Product : DotProduct  OutDataType=sfix(16)  OutScaling=2^-10  InputSameDT=on  OutDataTypeStr=Inherit: Inherit via internal rule
  Gain : Gain  Gain=Solar_Constant  ParameterDataType=sfix(16)  ParameterScaling=2^0  OutDataType=sfix(16)  OutScaling=2^0
  Gain1 : Gain  Gain=Area_SP_S6  ParameterDataType=sfix(16)  ParameterScaling=2^0  OutDataType=sfix(16)  OutScaling=2^0
  Product1 : Product  OutDataType=fixdt(1, 16)  OutScaling=2^0  RndMeth=Zero
  Saturation : Saturate  UpperLimit=1000  LowerLimit=0  OutDataType=fixdt(1, 16)  OutScaling=2^0
  Wattage in S6 : Outport  OutDataType=sfix(16)  OutScaling=2^0
  wires:
  v_Sunb/1 -> Dot Product/2
  Constant/1 -> Dot Product/1
  Gain1/1 -> Gain/1
  Gain/1 -> Wattage in S6/1
  Dot Product/1 -> Product1/1
  light1/1 -> Product1/2
  Product1/1 -> Saturation/1
  Saturation/1 -> Gain1/1

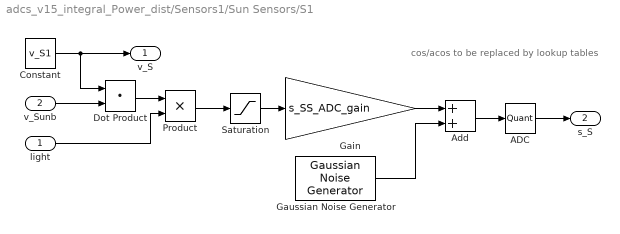
== system adcs_v15_integral_Power_dist/Sensors1/Sun Sensors/S1 ==
  note: cos/acos to be replaced by lookup tables
  light : Inport  OutDataType=sfix(16)  OutScaling=2^0
  v_Sunb : Inport  Port=2  OutDataType=sfix(16)  OutScaling=2^0
  ADC : Quantizer  QuantizationInterval=1/s_SS_ADC_res
  Add : Sum  OutDataType=sfix(16)  OutScaling=2^-10
  Constant : Constant  Value=v_S1  OutDataType=sfix(16)  OutScaling=2^0
  Dot Product : DotProduct  OutDataType=sfix(16)  OutScaling=2^-10  InputSameDT=on  OutDataTypeStr=Inherit: Inherit via internal rule
  Gain : Gain  Gain=s_SS_ADC_gain  ParameterDataType=sfix(16)  ParameterScaling=2^0  OutDataType=sfix(16)  OutScaling=2^0
  Gaussian Noise Generator : commnoisgen2/Gaussian Noise Generator  SystemSampleTime=-1  m=0  d=s_x_SUNSENSOR  s=41  Ts=s_SIM_STEP_SIZE  frameBased=off  sampPerFrame=1  orient=off  outDataType=double
  Product : Product  OutDataType=fixdt(1, 16)  OutScaling=2^0  RndMeth=Zero
  Saturation : Saturate  UpperLimit=inf  LowerLimit=0  OutDataType=sfix(16)  OutScaling=2^0
  v_S : Outport  OutDataType=sfix(16)  OutScaling=2^0
  s_S : Outport  Port=2  OutDataType=sfix(16)  OutScaling=2^0
  wires:
  light/1 -> Product/2
  Product/1 -> Saturation/1
  Dot Product/1 -> Product/1
  v_Sunb/1 -> Dot Product/2
  Saturation/1 -> Gain/1
  Constant/1 -> v_S/1, Dot Product/1
  Gaussian Noise Generator/1 -> Add/2
  Gain/1 -> Add/1
  Add/1 -> ADC/1
  ADC/1 -> s_S/1
